simulink model "dft_filter"  (R2021b)
settings: Solver=FixedStepDiscrete  StartTime=0.0  StopTime=10.0  FixedStep=0.001  RelTol=1e-3
values from neighbouring files (symbols this model uses):
  INJ_FREQ = 1.0    [dft_filter_dic.sldd]
  INJ_SAMPNUM = 1000.0    [dft_filter_dic.sldd]
  SAMP_FREQ = 1000.0    [dft_filter_dic.sldd]
settings Model: DataDictionary=dft_filter_dic.sldd  Creator=zqzq_  LastModifiedBy=zqzq_
settings OptimizationCC: DefaultParameterBehavior=Inlined  EnhancedBackFolding=on  PassReuseOutputArgsAs=Individual arguments  ZeroExternalMemoryAtStartup=off  ZeroInternalMemoryAtStartup=off  OptimizeBlockOrder=speed  DifferentSizesBufferReuse=on  OptimizationCustomize=off  EfficientTunableParamExpr=on
settings DebuggingCC: ParameterTunabilityLossMsg=error
settings SFSimCC: MATLABDynamicMemAlloc=off
settings RTWCC: Description=Embedded Coder  SystemTargetFile=ert.tlc  GenCodeOnly=on  TemplateMakefile=ert_default_tmf
settings CodeAppCC: ForceParamTrailComments=on  IgnoreCustomStorageClasses=off  OperatorAnnotations=on  SimulinkDataObjDesc=on  SFDataObjDesc=on  InsertBlockDesc=on
settings ERTTargetCC: TargetLangStandard=C99 (ISO)  GenerateSampleERTMain=on  InlinedParameterPlacement=NonHierarchical  ERTCustomFileTemplate=example_file_process.tlc

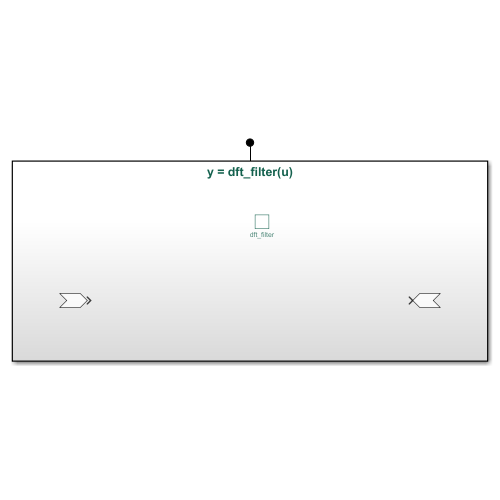
[thumbnail: Simulink's stored preview of the top-level diagram]
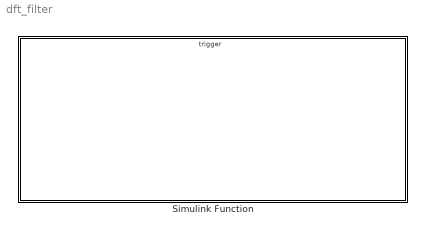
== system dft_filter ==
  Simulink Function : Subsystem  TreatAsAtomicUnit=on

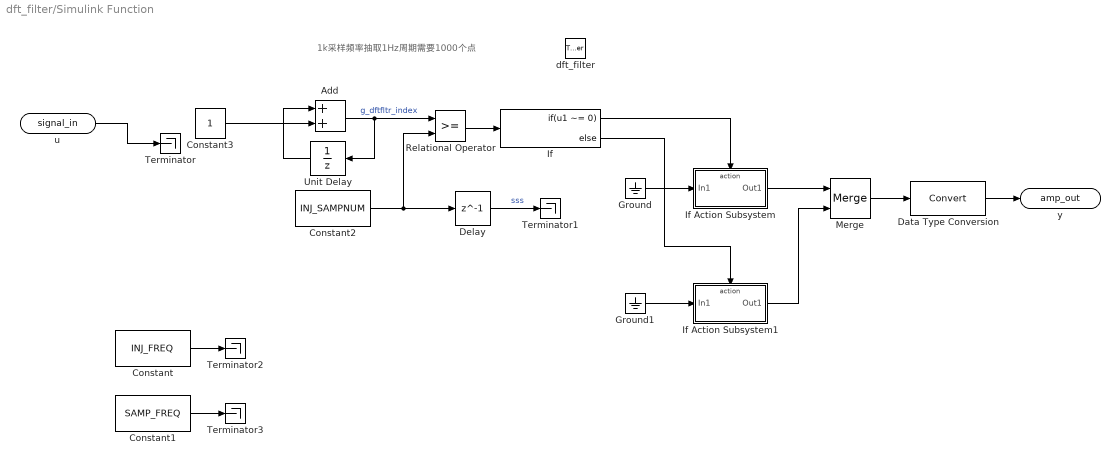
== system dft_filter/Simulink Function ==
  note: 1k采样频率抽取1Hz周期需要1000个点
  dft_filter : TriggerPort  TriggerType=function-call  IsSimulinkFunction=on  FunctionName=dft_filter_cal  VariantControl=(inherit)
  Add : Sum
  Constant : Constant  Value=INJ_FREQ
  Constant1 : Constant  Value=SAMP_FREQ
  Constant2 : Constant  Value=INJ_SAMPNUM
  Constant3 : Constant  OutDataTypeStr=uint16
  Data Type Conversion : DataTypeConversion
  Delay : Delay  DelayLength=1  InitialCondition=0
  Ground : Ground
  Ground1 : Ground
  If : If  IfExpression=u1 ~= 0
  If Action Subsystem : Subsystem  TreatAsAtomicUnit=on
  If Action Subsystem1 : Subsystem  TreatAsAtomicUnit=on
  Merge : Merge
  Relational Operator : RelationalOperator  OutDataTypeStr=boolean  RndMeth=Simplest
  Terminator{,1..3} (4 alike) : Terminator
  Unit Delay : UnitDelay  SampleTime=-1  HasFrameUpgradeWarning=on
  u : ArgIn  DisableCoverage=on  OutDataTypeStr=single  ArgumentName=signal_in
  y : ArgOut  DisableCoverage=on  OutDataTypeStr=single  ArgumentName=amp_out
  wires:
  If Action Subsystem/1(Out1) -> Merge/1
  If Action Subsystem1/1(Out1) -> Merge/2
  If/2 -> If Action Subsystem1/Action
  If/1 -> If Action Subsystem/Action
  Relational Operator/1 -> If/1
  Constant2/1 -> Delay/1, Relational Operator/2
  Add/1 -> Unit Delay/1, Relational Operator/1  "g_dftfltr_index"
  Constant3/1 -> Add/2
  u/1 -> Terminator/1
  Unit Delay/1 -> Add/1
  Constant/1 -> Terminator2/1
  Constant1/1 -> Terminator3/1
  Data Type Conversion/1 -> y/1
  Merge/1 -> Data Type Conversion/1
  Ground/1 -> If Action Subsystem/1(In1)
  Ground1/1 -> If Action Subsystem1/1(In1)
  Delay/1 -> Terminator1/1  "sss"

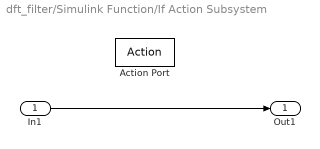
== system dft_filter/Simulink Function/If Action Subsystem ==
  In1 : Inport
  Action Port : ActionPort  ActionPortLabel=if(u1 ~= 0)
  Out1 : Outport
  wires:
  In1/1 -> Out1/1

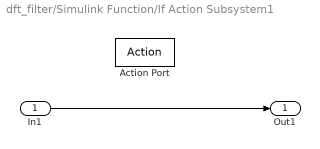
== system dft_filter/Simulink Function/If Action Subsystem1 ==
  In1 : Inport
  Action Port : ActionPort  ActionPortLabel=else
  Out1 : Outport
  wires:
  In1/1 -> Out1/1
